simulink model "ASW"  (R2020b)
settings: configuration reference "cs_ert" (kept outside this file)
settings Model: DataDictionary=ASW.sldd  Creator=zhoutinglin  LastModifiedBy=zhoutinglin
settings ConfigSetRef: SourceName=cs_ert

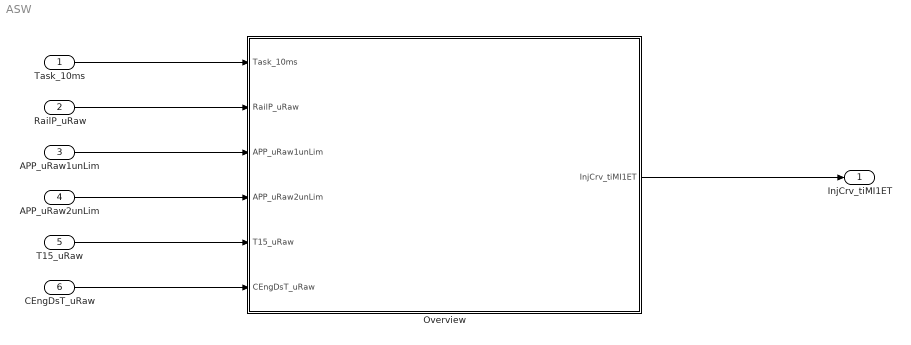
== system ASW ==
  Task_10ms : Inport  OutputFunctionCall=on
  RailP_uRaw : Inport  Port=2
  APP_uRaw1unLim : Inport  Port=3
  APP_uRaw2unLim : Inport  Port=4
  T15_uRaw : Inport  Port=5
  CEngDsT_uRaw : Inport  Port=6
  Overview : Subsystem
  InjCrv_tiMI1ET : Outport
  wires:
  Task_10ms/1 -> Overview/1(Task_10ms)
  RailP_uRaw/1 -> Overview/2(RailP_uRaw)
  APP_uRaw1unLim/1 -> Overview/3(APP_uRaw1unLim)
  APP_uRaw2unLim/1 -> Overview/4(APP_uRaw2unLim)
  T15_uRaw/1 -> Overview/5(T15_uRaw)
  CEngDsT_uRaw/1 -> Overview/6(CEngDsT_uRaw)
  Overview/1(InjCrv_tiMI1ET) -> InjCrv_tiMI1ET/1

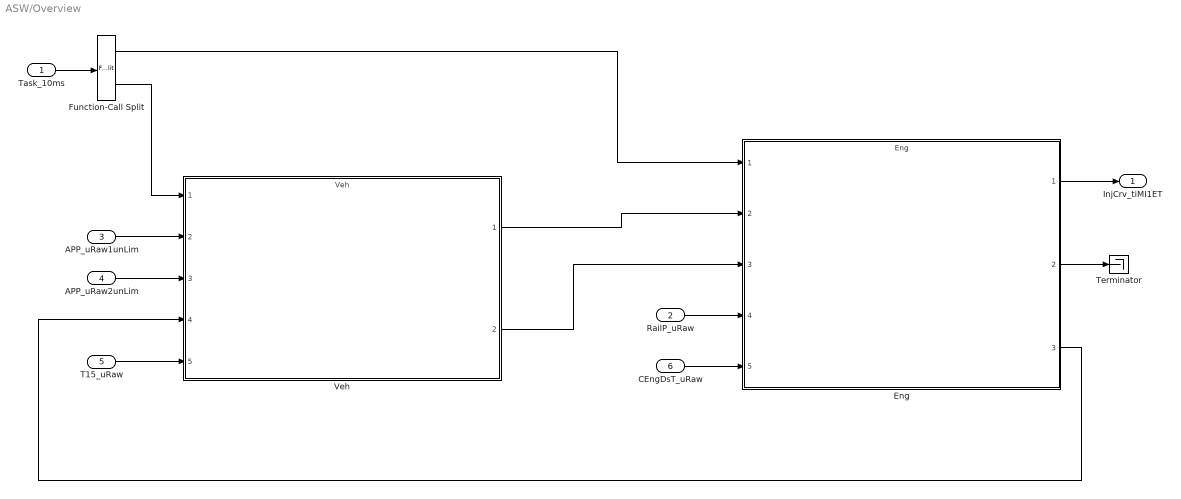
== system ASW/Overview ==
  Task_10ms : Inport
  RailP_uRaw : Inport  Port=2
  APP_uRaw1unLim : Inport  Port=3
  APP_uRaw2unLim : Inport  Port=4
  T15_uRaw : Inport  Port=5
  CEngDsT_uRaw : Inport  Port=6
  Eng : ModelReference  ModelNameDialog=Eng.slx  SimulationMode=Normal  ScheduleRates=on  ModelReferenceVersion=6.4
  Function-Call Split : FunctionCallSplit  IconShape=distinctive  NumOutputPorts=2  OutputPortLayout=default
  Terminator : Terminator
  Veh : ModelReference  ModelNameDialog=Veh  SimulationMode=Normal  ScheduleRates=on  ModelReferenceVersion=6.1
  InjCrv_tiMI1ET : Outport
  wires:
  Eng/1 -> InjCrv_tiMI1ET/1
  APP_uRaw1unLim/1 -> Veh/2
  APP_uRaw2unLim/1 -> Veh/3
  T15_uRaw/1 -> Veh/5
  Task_10ms/1 -> Function-Call Split/1
  Function-Call Split/2 -> Veh/1
  Function-Call Split/1 -> Eng/1
  RailP_uRaw/1 -> Eng/4
  CEngDsT_uRaw/1 -> Eng/5
  Veh/2 -> Eng/3
  Veh/1 -> Eng/2
  Eng/3 -> Veh/4
  Eng/2 -> Terminator/1
